simulink model "simulate_FM_Passband_v2"  (R2018a)
settings: Solver=VariableStepAuto  StartTime=0.0  StopTime=inf  RelTol=1e-3
libraries: simulink x2
settings Model: Creator=kelnhofer  LastModifiedBy=prust
settings CodeAppCC: StateflowObjectComments=on

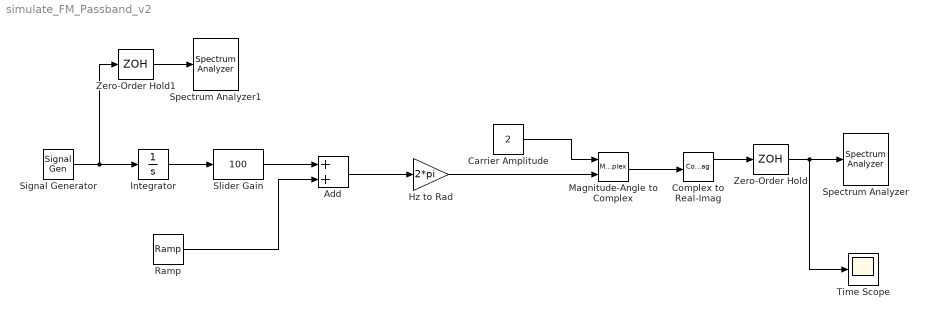
== system simulate_FM_Passband_v2 ==
  Add : Sum
  Carrier Amplitude : Constant  Value=2
  Complex to Real-Imag : ComplexToRealImag
  Hz to Rad : Gain  Gain=2*pi
  Integrator : Integrator
  Magnitude-Angle to Complex : MagnitudeAngleToComplex
  Ramp : simulink/Sources/Ramp  slope=1000  start=0  InitialOutput=0
  Signal Generator : SignalGenerator  Frequency=10
  Slider Gain : simulink/Math Operations/Slider Gain  gain=100  low=0  high=600
  Spectrum Analyzer : SpectrumAnalyzer
  Spectrum Analyzer1 : SpectrumAnalyzer
  Time Scope : Scope
  Zero-Order Hold : ZeroOrderHold  SampleTime=1/8000
  Zero-Order Hold1 : ZeroOrderHold  SampleTime=1/8000
  wires:
  Carrier Amplitude/1 -> Magnitude-Angle to Complex/1
  Add/1 -> Hz to Rad/1
  Magnitude-Angle to Complex/1 -> Complex to Real-Imag/1
  Complex to Real-Imag/1 -> Zero-Order Hold/1
  Signal Generator/1 -> Zero-Order Hold1/1, Integrator/1
  Integrator/1 -> Slider Gain/1
  Ramp/1 -> Add/2
  Zero-Order Hold/1 -> Spectrum Analyzer/1, Time Scope/1
  Hz to Rad/1 -> Magnitude-Angle to Complex/2
  Slider Gain/1 -> Add/1
  Zero-Order Hold1/1 -> Spectrum Analyzer1/1
